simulink model "controlHibrido_ESTE"  (R2018a)
settings: Solver=FixedStepAuto  StartTime=0.0  StopTime=10  FixedStep=0.01  RelTol=1e-3
values from neighbouring files (symbols this model uses):
  fd = 10    [ctrl_fuerza.m]
  Kenv = 1e3    (= 1000)    [ctrl_fuerza.m]
  kp = 25    [Calculo_Tau_RR.m]
  kpf = 144    [ctrl_fuerza.m]
  kv = 2*sqrt(kp)    [Calculo_Tau_RR.m]
  kvf = 2*sqrt(kpf)    [ctrl_fuerza.m]
  R_Pared_Cart = [cos(pi/4) sin(pi/4);-sin(pi/4) cos(pi/4)]    [ctrl_fuerza.m]
  theta0_1 = -20.53*pi/180    (= -0.358316095434)    [ctrl_fuerza.m]
  theta0_2 = pi/4 +abs(theta0_1)    [ctrl_fuerza.m]
libraries: roblocks x16, simulink x1
settings Model: Creator=Marcelo  LastModifiedBy=Marcelo
settings DataIOCC: ReturnWorkspaceOutputs=on
settings SFSimCC: SimUseLocalCustomCode=on
settings RTWCC: RTWUseLocalCustomCode=on

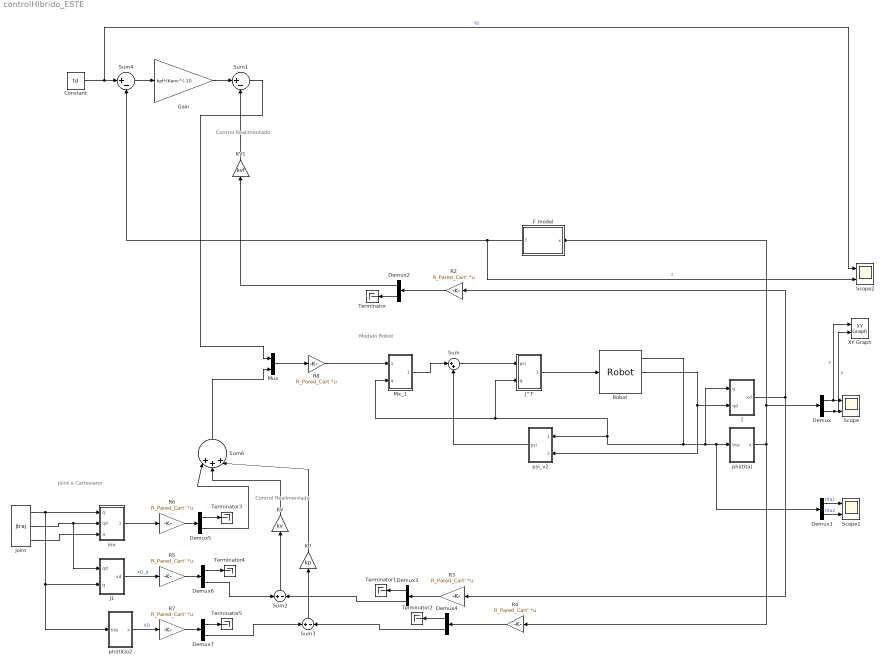
== system controlHibrido_ESTE ==
  note: Control Realimentado
  note: Control Realimentado
  note: Modelo Robot
  note: Joint a Cartesiano
  Constant : Constant  Value=fd
  Demux{,1..7} (8 alike) : Demux  Outputs=2
  "F model " : MATLAB Function  TreatAsAtomicUnit=on
  Gain : Gain  Gain=kpf*(Kenv^(-1))
  J : Subsystem
  J1 : Subsystem
  J^T : Subsystem
  KP : Gain  Gain=kp
  KV : Gain  Gain=kv
  KV1 : Gain  Gain=kvf
  Mux : Mux  Inputs=2
  Mx_1 : Subsystem
  R{2..7} (6 alike) : Gain  Gain=R_Pared_Cart'  Multiplication=Matrix(K*u)
  R8 : Gain  Gain=R_Pared_Cart  Multiplication=Matrix(K*u)
  Robot : roblocks/Arm/Robot  robot=Robot  q0=[theta0_1 theta0_2]
  Scope : Scope  NumInputPorts=2
  Scope1 : Scope  NumInputPorts=2
  Scope2 : Scope  NumInputPorts=2
  Sum : Sum  Inputs=|++
  Sum1 : Sum  Inputs=|+-
  Sum2 : Sum  Inputs=+|-
  Sum3 : Sum  Inputs=+|-
  Sum4 : Sum  Inputs=|+-
  Sum6 : Sum  Inputs=|+++|
  Terminator{,1..5} (6 alike) : Terminator
  XY Graph : simulink/Sinks/XY Graph  xmin=0  xmax=2  ymin=0  ymax=2  st=-1
  inv : Subsystem
  joint : roblocks/Toolbox/jtraj  q0=[theta0_1 theta0_2]  qf=[0 pi/2]  tmax=5  ts=0.02
  phi(tita) : Subsystem
  phi(tita)2 : Subsystem
  psi_v2 : Subsystem
  wires:
  Sum2/1 -> KV/1
  Sum3/1 -> KP/1
  Sum4/1 -> Gain/1
  Gain/1 -> Sum1/1
  "F model "/1(f) -> Scope2/2, Sum4/2  "f"
  KV1/1 -> Sum1/2
  KP/1 -> Sum6/3
  Constant/1 -> Scope2/1, Sum4/1  "fd"
  Demux1/1 -> Scope1/1  "tita1"
  Demux1/2 -> Scope1/2  "tita2"
  Demux/2 -> XY Graph/2, Scope/2  "y"
  Demux/1 -> XY Graph/1, Scope/1  "x"
  J^T/1(tau) -> Robot/1
  Sum/1 -> J^T/1(psi)
  Robot/1 -> J/1(q), Demux1/1, phi(tita)/1(tita), psi_v2/1(tita), Mx_1/2(q), J^T/2(q)
  Robot/2 -> psi_v2/2(tita_d), J/2(qd)
  phi(tita)/1(x) -> R4/1, Demux/1, "F model "/1(x)
  J/1(xd) -> R2/1, R3/1
  KV/1 -> Sum6/2
  joint/3 -> inv/3(qdd)
  joint/2 -> J1/1(qd), inv/2(qd)
  joint/1 -> inv/1(q), J1/2(q), phi(tita)2/1(tita)
  psi_v2/1(psi) -> Sum/2
  Mx_1/1(psi_o) -> Sum/1
  R2/1 -> Demux2/1
  Demux2/1 -> KV1/1
  Demux2/2 -> Terminator/1
  Sum1/1 -> Mux/1
  R4/1 -> Demux4/1
  R3/1 -> Demux3/1
  Demux3/2 -> Sum2/2
  Demux4/2 -> Sum3/2
  Demux4/1 -> Terminator2/1
  Demux3/1 -> Terminator1/1
  phi(tita)2/1(x) -> R7/1  "XD"
  J1/1(xd) -> R5/1  "XD_d"
  inv/1(xdd) -> R6/1
  R6/1 -> Demux5/1
  R5/1 -> Demux6/1
  R7/1 -> Demux7/1
  Demux5/2 -> Sum6/1
  Demux6/2 -> Sum2/1
  Demux7/2 -> Sum3/1
  Demux5/1 -> Terminator3/1
  Demux6/1 -> Terminator4/1
  Demux7/1 -> Terminator5/1
  Sum6/1 -> Mux/2
  R8/1 -> Mx_1/1(x_dd)
  Mux/1 -> R8/1

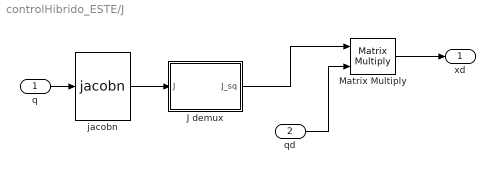
== system controlHibrido_ESTE/J ==
  q : Inport
  qd : Inport  Port=2
  J demux : MATLAB Function  TreatAsAtomicUnit=on
  Matrix Multiply : Product  Multiplication=Matrix(*)
  jacobn : roblocks/Arm/jacobn  robot=Robot
  xd : Outport
  wires:
  jacobn/1 -> J demux/1(J)
  qd/1 -> Matrix Multiply/2
  q/1 -> jacobn/1
  J demux/1(J_sq) -> Matrix Multiply/1
  Matrix Multiply/1 -> xd/1

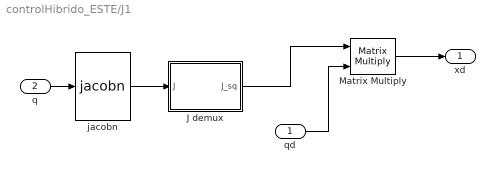
== system controlHibrido_ESTE/J1 ==
  qd : Inport
  q : Inport  Port=2
  J demux : MATLAB Function  TreatAsAtomicUnit=on
  Matrix Multiply : Product  Multiplication=Matrix(*)
  jacobn : roblocks/Arm/jacobn  robot=Robot
  xd : Outport
  wires:
  jacobn/1 -> J demux/1(J)
  qd/1 -> Matrix Multiply/2
  q/1 -> jacobn/1
  J demux/1(J_sq) -> Matrix Multiply/1
  Matrix Multiply/1 -> xd/1

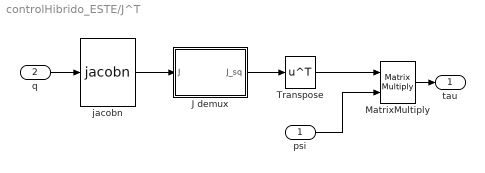
== system controlHibrido_ESTE/J^T ==
  psi : Inport
  q : Inport  Port=2
  J demux : MATLAB Function  TreatAsAtomicUnit=on
  MatrixMultiply : Product  Multiplication=Matrix(*)
  Transpose : Math  Operator=transpose  SaturateOnIntegerOverflow=on
  jacobn : roblocks/Arm/jacobn  robot=Robot
  tau : Outport
  wires:
  MatrixMultiply/1 -> tau/1
  q/1 -> jacobn/1
  jacobn/1 -> J demux/1(J)
  J demux/1(J_sq) -> Transpose/1
  Transpose/1 -> MatrixMultiply/1
  psi/1 -> MatrixMultiply/2

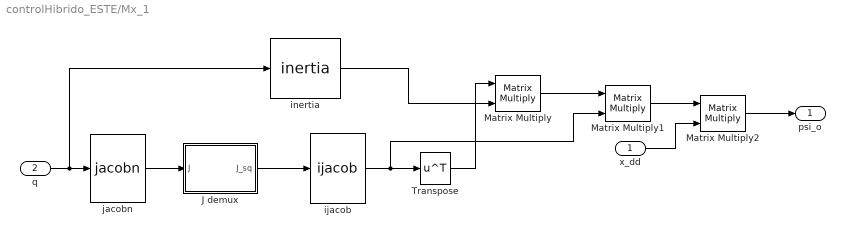
== system controlHibrido_ESTE/Mx_1 ==
  x_dd : Inport
  q : Inport  Port=2
  J demux : MATLAB Function  TreatAsAtomicUnit=on
  Matrix Multiply : Product  Multiplication=Matrix(*)
  Matrix Multiply1 : Product  Multiplication=Matrix(*)
  Matrix Multiply2 : Product  Multiplication=Matrix(*)
  Transpose : Math  Operator=transpose  SaturateOnIntegerOverflow=on
  ijacob : roblocks/Arm/ijacob
  inertia : roblocks/Arm/inertia  robot=Robot
  jacobn : roblocks/Arm/jacobn  robot=Robot
  psi_o : Outport
  wires:
  ijacob/1 -> Matrix Multiply1/2, Transpose/1
  Matrix Multiply1/1 -> Matrix Multiply2/1
  q/1 -> inertia/1, jacobn/1
  Transpose/1 -> Matrix Multiply/1
  J demux/1(J_sq) -> ijacob/1
  Matrix Multiply/1 -> Matrix Multiply1/1
  Matrix Multiply2/1 -> psi_o/1
  jacobn/1 -> J demux/1(J)
  x_dd/1 -> Matrix Multiply2/2
  inertia/1 -> Matrix Multiply/2

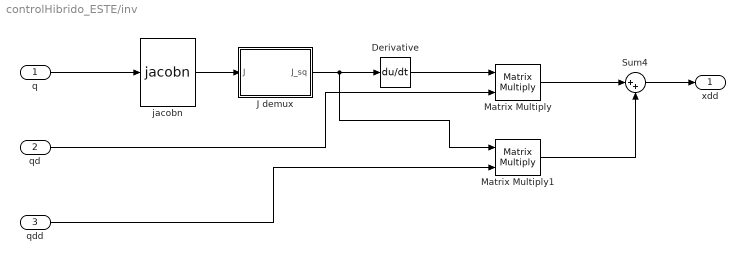
== system controlHibrido_ESTE/inv ==
  q : Inport
  qd : Inport  Port=2
  qdd : Inport  Port=3
  Derivative : Derivative
  J demux : MATLAB Function  TreatAsAtomicUnit=on
  Matrix Multiply : Product  Multiplication=Matrix(*)
  Matrix Multiply1 : Product  Multiplication=Matrix(*)
  Sum4 : Sum  Inputs=|++
  jacobn : roblocks/Arm/jacobn  robot=Robot
  xdd : Outport
  wires:
  Matrix Multiply/1 -> Sum4/1
  q/1 -> jacobn/1
  J demux/1(J_sq) -> Matrix Multiply1/1, Derivative/1
  Matrix Multiply1/1 -> Sum4/2
  qd/1 -> Matrix Multiply/2
  Sum4/1 -> xdd/1
  qdd/1 -> Matrix Multiply1/2
  jacobn/1 -> J demux/1(J)
  Derivative/1 -> Matrix Multiply/1

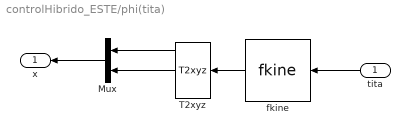
== system controlHibrido_ESTE/phi(tita) ==
  tita : Inport
  Mux : Mux  Inputs=2
  T2xyz : roblocks/Toolbox/T2xyz
  fkine : roblocks/Arm/fkine  robot=Robot
  x : Outport
  wires:
  T2xyz/2 -> Mux/2
  Mux/1 -> x/1
  fkine/1 -> T2xyz/1
  tita/1 -> fkine/1
  T2xyz/1 -> Mux/1

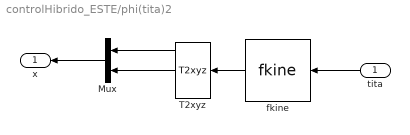
== system controlHibrido_ESTE/phi(tita)2 ==
  tita : Inport
  Mux : Mux  Inputs=2
  T2xyz : roblocks/Toolbox/T2xyz
  fkine : roblocks/Arm/fkine  robot=Robot
  x : Outport
  wires:
  T2xyz/2 -> Mux/2
  Mux/1 -> x/1
  fkine/1 -> T2xyz/1
  tita/1 -> fkine/1
  T2xyz/1 -> Mux/1

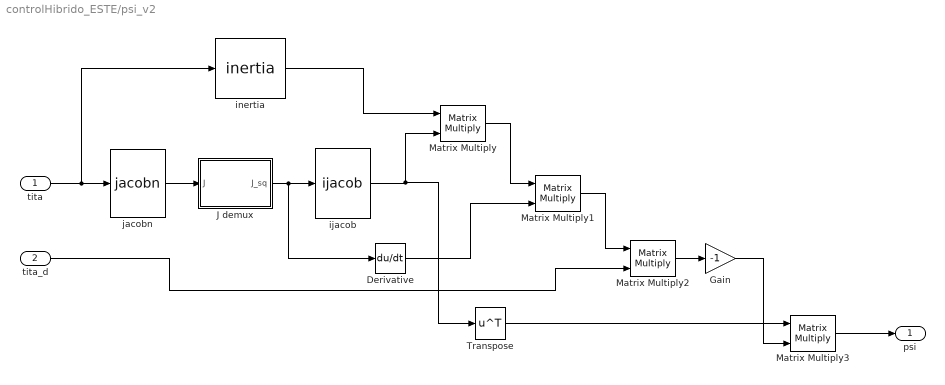
== system controlHibrido_ESTE/psi_v2 ==
  tita : Inport
  tita_d : Inport  Port=2
  Derivative : Derivative
  Gain : Gain  Gain=-1
  J demux : MATLAB Function  TreatAsAtomicUnit=on
  Matrix Multiply{,1..3} (4 alike) : Product  Multiplication=Matrix(*)
  Transpose : Math  Operator=transpose  SaturateOnIntegerOverflow=on
  ijacob : roblocks/Arm/ijacob
  inertia : roblocks/Arm/inertia  robot=Robot
  jacobn : roblocks/Arm/jacobn  robot=Robot
  psi : Outport
  wires:
  inertia/1 -> Matrix Multiply/1
  Matrix Multiply/1 -> Matrix Multiply1/1
  tita/1 -> inertia/1, jacobn/1
  tita_d/1 -> Matrix Multiply2/2
  ijacob/1 -> Transpose/1, Matrix Multiply/2
  J demux/1(J_sq) -> Derivative/1, ijacob/1
  Derivative/1 -> Matrix Multiply1/2
  jacobn/1 -> J demux/1(J)
  Matrix Multiply1/1 -> Matrix Multiply2/1
  Matrix Multiply3/1 -> psi/1
  Transpose/1 -> Matrix Multiply3/1
  Matrix Multiply2/1 -> Gain/1
  Gain/1 -> Matrix Multiply3/2

== matlab function controlHibrido_ESTE/J^T/J demux ==
  data: J input; J_sq output
function J_sq = fcn(J)

J_sq = [J(1,1) J(1,2);J(2,1) J(2,2)];

== matlab function controlHibrido_ESTE/F model  ==
  data: x input; f output
function f = fcn(x)
p1 = [0; 2];
p2 = [2; 0];

% checkeo de que lado de la pared esta el punto
% https://stackoverflow.com/questions/3838319/how-can-i-check-if-a-point-is-below-a-line-or-not
v1 = p2-p1;  % v1 = [2, -2] siempre
v2 = p2-x;   % v2 = [2-x, -y]
cross_prod = v1(1)*v2(2)-v1(2)*v2(1);
% ejemplo: si (x,y) = (0, 0), v2=[2, 0] y cross_prod=2*0+2*2=+4 > 0
% entonces el lado en el que estoy "adentro de la pared"
% es el que corresponde a cross(v1, v2) < 0
if cross_prod < 0
    K_env = 1e3; % 1000N/mm = 1e6N/m
    ke = diag([cos(pi/4)*K_env, sin(pi/4)*K_env]);
    % calculo del punto mas cercano a x sobre la recta ax+by+c=0
    % nuestra recta es x+y-2=0
    a = 1;
    b = 1;
    c = -2;
    x0 = x(1); y0 = x(2);
    xp1 = (b*(b*x0-a*y0)-a*c) / (a^2+b^2);
    xp2 = (a*(-b*x0+a*y0)-b*c) / (a^2+b^2);
    xp = [xp1; xp2];

    f = K_env * norm(x - xp);
else
    f = 0;
end

% 
% % distancia de un punto a una linea definida por dos puntos:
% % https://en.wikipedia.org/wiki/Distance_from_a_point_to_a_line
% 
% % esto podria simplificarse porque hay terminos que son 0, pero asi queda
% % generico para cualquier pared
% num = abs( (p2(2)-p1(2))*x(1) - (p2(1)-p1(1))*x(2)...
%     + p2(1)*p1(2) - p2(2)*p1(1) );
% % el denominador es la distancia entre los dos puntos que definen la linea
% den = dist(p1, p2);
% d = num/den;

== matlab function controlHibrido_ESTE/J1/J demux ==
  data: J input; J_sq output
function J_sq = fcn(J)

J_sq = [J(1,1) J(1,2);J(2,1) J(2,2)];

== matlab function controlHibrido_ESTE/Mx_1/J demux ==
  data: J input; J_sq output
function J_sq = fcn(J)

J_sq = [J(1,1) J(1,2);J(2,1) J(2,2)];

== matlab function controlHibrido_ESTE/J/J demux ==
  data: J input; J_sq output
function J_sq = fcn(J)

J_sq = [J(1,1) J(1,2);J(2,1) J(2,2)];

== matlab function controlHibrido_ESTE/psi_v2/J demux ==
  data: J input; J_sq output
function J_sq = fcn(J)

J_sq = [J(1,1) J(1,2);J(2,1) J(2,2)];

== matlab function controlHibrido_ESTE/inv/J demux ==
  data: J input; J_sq output
function J_sq = fcn(J)

J_sq = [J(1,1) J(1,2);J(2,1) J(2,2)];
